simulink model "zynq_pmsm_motor_control"  (R2019b)
settings: Solver=FixedStepDiscrete  StartTime=0.0  StopTime=5000  FixedStep=0.002  RelTol=1e-3  EnableMultiTasking=on
undefined symbols (not defined in the file): DiscIntNeverNeededParam
libraries: simulink x1, simulink_extras x1
settings Model: SimulationMode=external  ExtModeTrigDuration=200000  Creator=krecmich  LastModifiedBy=cernylu6
settings DataIOCC: LimitDataPoints=on  SaveFormat=Array
settings OptimizationCC: ExpressionDepthLimit=2147483647  LifeSpan=1  EfficientTunableParamExpr=on
settings DebuggingCC: UnderspecifiedInitializationDetection=Classic  MergeDetectMultiDrivingBlocksExec=none  SolverPrmCheckMsg=warning  StateNameClashWarn=warning  SFUnexpectedBacktrackingDiag=warning  SFNoUnconditionalDefaultTransitionDiag=warning  SFExecutionAtInitializationDiag=none  ArithmeticOperatorsInVariantConditions=warning
settings HardwareCC: ProdBitPerLong=64  ProdLargestAtomicFloat=None  ProdHWDeviceType=Intel->x86-64
settings ModelReferenceCC: PropagateSignalLabelsOutOfModel=off
settings SFSimCC: SimUseLocalCustomCode=off  MATLABDynamicMemAlloc=off  CustomCodeUndefinedFunction=UseInterfaceOnly
settings RTWCC: Description=Linux Embedded Coder  SystemTargetFile=ert_linux.tlc  MakeCommand="make_rtw OPT_OPTS=\"-O2 -ggdb -Wall\" CC=arm-linux-gnueabihf-gcc CPP=arm-linux-gnueabihf-gcc"  TemplateMakefile=ert_linux.tmf  RTWUseLocalCustomCode=off  CustomSource=zynq_3pmdrv1_mc.c
settings CodeAppCC: IgnoreCustomStorageClasses=off  CustomSymbolStrType=$N$R$M  StateflowObjectComments=on  InternalIdentifier=Classic
settings STFCustomTargetCC: TargetLangStandard=C99 (ISO)  ModelReferenceCompliant=off  CombineOutputUpdateFcns=on  ERTCustomFileBanners=on  RemoveResetFunc=on  MATLABClassNameForMDSCustomization=Simulink.SoftwareTarget.ERTCustomization  SystemTargetFile=ert_linux.tlc
settings ERTTargetCC: TargetLangStandard=C99 (ISO)  MultiwordLength=2048  ModelReferenceCompliant=off  ParMdlRefBuildCompliant=off  CompOptLevelCompliant=off  ConcurrentExecutionCompliant=off  SupportContinuousTime=on  SupportNonInlinedSFcns=on  ModelStepFunctionPrototypeControlCompliant=off  CPPClassGenCompliant=off  UseToolchainInfoCompliant=off  ExtMode=on  ExtModeMexArgs='192.168.136.74'  ERTCustomFileTemplate=ert_linux_file_process.tlc  ConvertIfToSwitch=off  SuppressUnreachableDefaultCases=off
settings ConfigComp: CovMetricSettings=dw  CovHtmlReporting=on  CovSaveCumulativeToWorkspaceVar=on  CovSaveSingleToWorkspaceVar=on  CovExternalEMLEnable=off

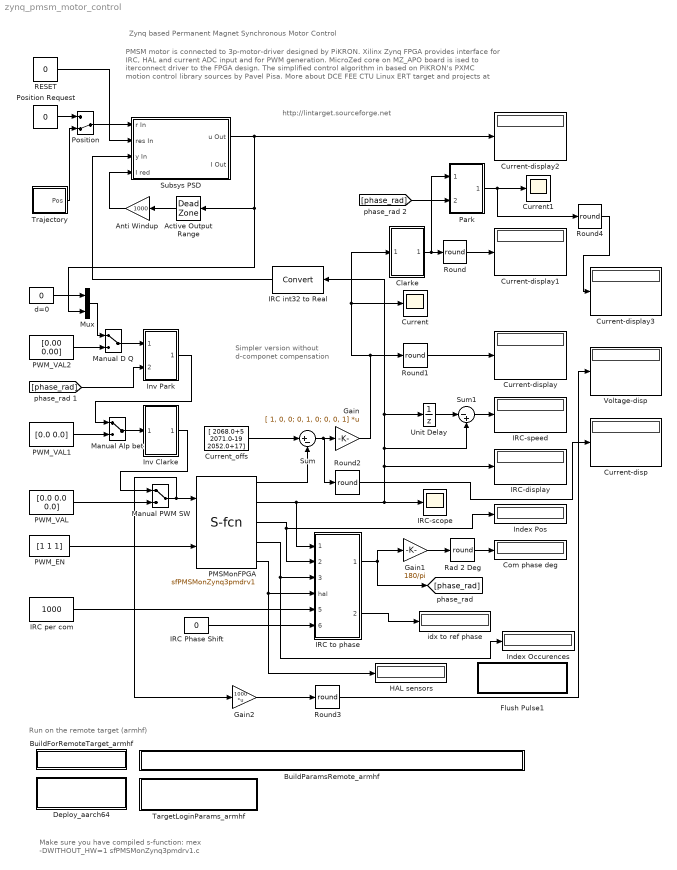
== system zynq_pmsm_motor_control ==
  note: Make sure you have compiled s-function:
      | mex -DWITHOUT_HW=1 sfPMSMonZynq3pmdrv1.c
  note: Simpler version without
      | d-componet compensation
  note: http://lintarget.sourceforge.net
  note: PMSM motor is connected to 3p-motor-driver designed by PiKRON. Xilinx Zynq FPGA provides
      | interface for  IRC, HAL and current ADC input and for PWM generation.
      | MicroZed core on MZ_APO board is ised to iterconnect driver to the FPGA design.
      | The simplified control algorithm in based on PiKRON's PXMC motion control
      | library sources by Pavel Pisa. More about DCE FEE CTU Linux ERT target and projects at
  note: Zynq based Permanent Magnet Synchronous Motor Control
  note: Run on the remote target (armhf)
  "  RESET" : Constant  Value=0
      settings: OpenFcn=if get_param(gcbh,'value')=='0' set_param(gcbh,'value','1'); else set_param(gcbh,'value','0'); end;
  Active Output Range : DeadZone  LowerValue=-0.8  UpperValue=0.8  LinearizeAsGain=off
  Anti Windup : Gain  Gain=1000
  BuildForRemoteTarget_armhf : Subsystem
      settings: OpenFcn=ert_linux_build(gcs, 'BuildParamsRemote_armhf')
      mask Display: disp('Build')
  BuildParamsRemote_armhf : Subsystem  mask{make_command='make_rtw OPT_OPTS="-O2 -ggdb -Wall" CC=arm-linux-gnueabihf-gcc CPP=arm-linux-gnueabihf-gcc'}
      mask prompts: make_command "MakeCommand"
      mask Display: disp(get_param(gcb, 'make_command'));
  Clarke : Subsystem
  Com phase deg : Display
  Current : Scope
  Current-disp : Display
  Current-display{,1..3} (4 alike) : Display
  Current1 : Scope
  Current_offs : Constant  Value="[ 2068.0+5  2071.0-19  2052.0+17]"
  Deploy_aarch64 : Subsystem
      settings: OpenFcn=ert_linux_deploy_and_connect(gcs, 'TargetLoginParams_armhf');
      mask Display: disp('Deploy and\nconnect')
  Flush Pulse1 : Subsystem  mask{target_ip_address='192.168.3.37'}
      mask prompts: target_ip_address "Target IP address"
      settings: OpenFcn=system(['./run_model_pmsm.sh ', get_param(bdroot(gcbh),'name'),' ', get_param(gcbh,'target_ip_address')]);
      mask Display: disp('Double Click\n to run model on Zynq')
  Gain : Gain  Gain=[ 1, 0, 0; 0, 1, 0; 0, 0, 1]  Multiplication=Matrix(K*u)
  Gain1 : Gain  Gain=180/pi
  Gain2 : Gain  Gain=1000  Multiplication=Matrix(K*u)
  HAL sensors : Display
  IRC Phase Shift : Constant  Value=0
  IRC int32 to Real : DataTypeConversion
  IRC per com : Constant  Value=1000  OutDataTypeStr=uint32
  IRC to phase : Subsystem
  IRC-display : Display
  IRC-scope : Scope
  IRC-speed : Display
  Index Occurences : Display
  Index Pos : Display
  Inv Clarke : Subsystem
  Inv Park : Subsystem
  Manual Alp bet : ManualSwitch
  Manual D Q : ManualSwitch
  Manual PWM SW : ManualSwitch
  Mux : Mux  Inputs=2
  PMSMonFPGA : S-Function  FunctionName=sfPMSMonZynq3pmdrv1  Parameters=Ts  SFunctionDeploymentMode=off  EnableBusSupport=off  mask{Ts=0.002}
      mask prompts: Ts "Sampling period (Ts):"
  PWM_EN : Constant  Value=[1 1 1]
  PWM_VAL : Constant  Value=[0.0 0.0 0.0]
  PWM_VAL1 : Constant  Value=[0.0 0.0]
  PWM_VAL2 : Constant  Value=[0.00 0.00]
  Park : Subsystem
  Position : ManualSwitch  CurrentSetting=0
  Position Request : Constant  Value=0
  Rad 2 Deg : Rounding  Operator=round
  Round{,1..4} (5 alike) : Rounding  Operator=round
  Subsys PSD : Subsystem  mask(optimized PSD controller){P=0.0006, I=0.002, D=0.001, Ts=0.002}
      mask prompts: P "P proportional (P):"; I "I integral (I):"; D "D derivative (D):"; Ts "Sampling period (Ts):"
      mask help:
      | Type: Subsystem block.
      |
      | Description:
      |   Subsystem covers optimized PSD controller (PSD represents discretized PID).
      |
      | Requirements:
      |   Sampling period Ts.
      mask Help:
      | <b>Type:</b> Subsystem block.
      | <br><br>
      | <b>Description:</b><br>
      |   Subsystem covers optimized PSD controller (PSD represents discretized PID).
      | <br><br>
      | <b>Requirements:</b><br>
      |   Sampling period Ts.
      mask Display:
      | color('orange');disp('\n          Opt. PSD\n          Controller');
      | color('green');port_label('input', 1, 'w');
      | color('red');port_label('input', 2, ' RSTs');
      | color('lightblue');port_label('input', 3, 'r');
      | color('orange');port_label('input', 4, 'red I');
      | color('orange');port_label('output', 1, 'u ');
      | color('orange');port_label('output', 2, 'I  ');
      | color('red');disp('\n\n\n\n\n\n\n       P');
  Sum : Sum  Inputs=|+-
  Sum1 : Sum  Inputs=|-+
  TargetLoginParams_armhf : Subsystem  mask{trgt_ip_addr='192.168.136.74', trgt_username='root'}
      mask prompts: trgt_ip_addr "Target IP address"; trgt_username "Target username"
      mask Display:
      | ip_addr = get_param(gcb, 'trgt_ip_addr');
      | user = get_param(gcb, 'trgt_username');
      | 
      | fprintf('IP addr:\t %s\n User:\t %s ', ip_addr, user);
  Trajectory : Subsystem
  Unit Delay : UnitDelay  SampleTime=-1  HasFrameUpgradeWarning=on
  Voltage-disp : Display
  d=0 : Constant  Value=0
  idx to ref phase : Display
  wires:
  Subsys PSD/1(u Out) -> Mux/2, Active Output Range/1, Current-display2/1
  "  RESET"/1 -> Subsys PSD/2(res In)
  Active Output Range/1 -> Anti Windup/1
  Anti Windup/1 -> Subsys PSD/4(I red)
  Position/1 -> Subsys PSD/1(r In)
  Position Request/1 -> Position/1
  Trajectory/1(Pos) -> Position/2
  PMSMonFPGA/2 -> IRC-scope/1, Unit Delay/1, IRC int32 to Real/1, Sum1/2, IRC-display/1, IRC to phase/1(irc_val)
  PWM_EN/1 -> PMSMonFPGA/2
  Round1/1 -> Current-display/1
  Current_offs/1 -> Sum/1
  Gain/1 -> Clarke/1("a, b, c"), Current/1, Round1/1
  PWM_VAL/1 -> Manual PWM SW/2
  Manual PWM SW/1 -> Gain2/1, PMSMonFPGA/1
  Round/1 -> Current-display1/1
  Clarke/1("alp, bet") -> Park/1("alp, bet"), Round/1
  PWM_VAL1/1 -> Manual Alp bet/2
  Manual Alp bet/1 -> Inv Clarke/1(alp,bet)
  Inv Clarke/1(a,b,c) -> Manual PWM SW/1
  Inv Park/1(alp,bet) -> Manual Alp bet/1
  Manual D Q/1 -> Inv Park/1(d,q)
  PWM_VAL2/1 -> Manual D Q/2
  Mux/1 -> Manual D Q/1
  d=0/1 -> Mux/1
  IRC to phase/1(phase rad) -> Gain1/1, [phase_rad]
  [phase_rad] -> Inv Park/2(angle rad)
  Gain1/1 -> Rad 2 Deg/1
  Rad 2 Deg/1 -> Com phase deg/1
  PMSMonFPGA/5 -> HAL sensors/1, IRC to phase/4(hal)
  IRC per com/1 -> IRC to phase/5(irc_per_com)
  PMSMonFPGA/3 -> Index Pos/1, IRC to phase/2(irc_indx)
  PMSMonFPGA/4 -> IRC to phase/3(irc_occur), Index Occurences/1
  [phase_rad] -> Park/2(angle rad)
  Park/1("d, q") -> Round4/1, Current1/1
  Unit Delay/1 -> Sum1/1
  Sum1/1 -> IRC-speed/1
  IRC int32 to Real/1 -> Subsys PSD/3(y In)
  IRC Phase Shift/1 -> IRC to phase/6(irc_ph_shift)
  Round2/1 -> Current-disp/1
  Gain2/1 -> Round3/1
  Round3/1 -> Voltage-disp/1
  Sum/1 -> Round2/1, Gain/1
  Round4/1 -> Current-display3/1
  PMSMonFPGA/1 -> Sum/2
  IRC to phase/2(idx to ref phase) -> idx to ref phase/1

== system zynq_pmsm_motor_control/BuildForRemoteTarget_armhf ==

== system zynq_pmsm_motor_control/BuildParamsRemote_armhf ==

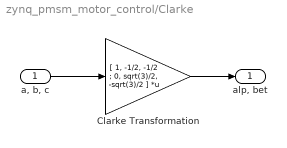
== system zynq_pmsm_motor_control/Clarke ==
  "a, b, c" : Inport
  Clarke Transformation : Gain  Gain=[ 1, -1/2, -1/2 ; 0, sqrt(3)/2, -sqrt(3)/2 ]  Multiplication=Matrix(K*u)
  "alp, bet" : Outport
  wires:
  "a, b, c"/1 -> Clarke Transformation/1
  Clarke Transformation/1 -> "alp, bet"/1

== system zynq_pmsm_motor_control/Deploy_aarch64 ==

== system zynq_pmsm_motor_control/Flush Pulse1 ==

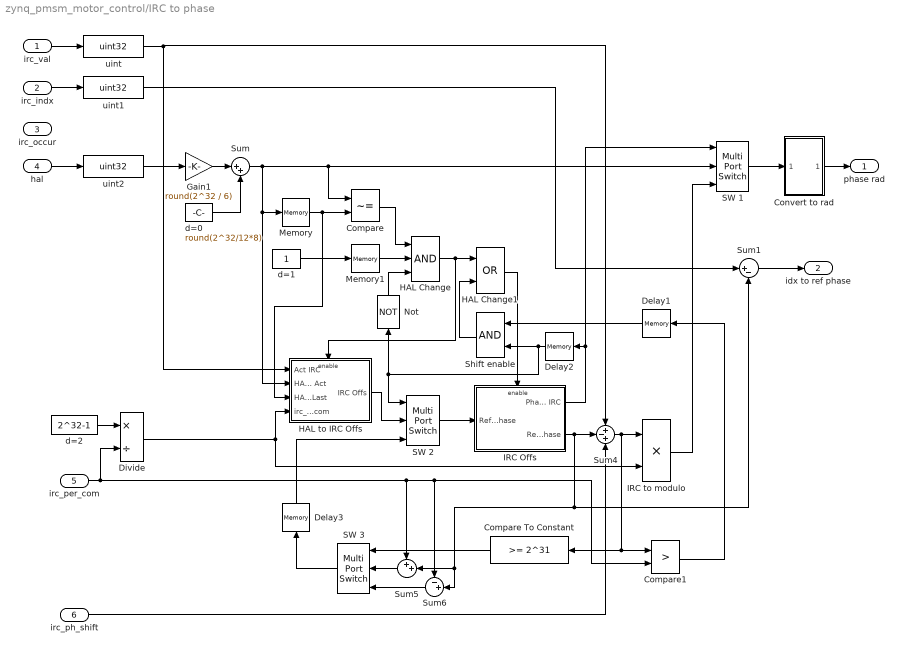
== system zynq_pmsm_motor_control/IRC to phase ==
  irc_val : Inport
  irc_indx : Inport  Port=2
  irc_occur : Inport  Port=3
  hal : Inport  Port=4
  irc_per_com : Inport  Port=5
  irc_ph_shift : Inport  Port=6
  Compare : RelationalOperator  Operator=~=  OutDataTypeStr=boolean  RndMeth=Nearest  InputSameDT=on
  Compare To Constant : simulink/Logic and Bit Operations/Compare To Constant  relop=>=  const=2^31  OutDataTypeStr=boolean
  Compare1 : RelationalOperator  Operator=>  OutDataTypeStr=boolean  RndMeth=Nearest  InputSameDT=on
  Convert to rad : Subsystem
  Delay1 : Memory
  Delay2 : Memory
  Delay3 : Memory
  Divide : Product  Inputs=*/  OutDataTypeStr=uint32
  Gain1 : Gain  Gain=round(2^32 / 6)  OutDataTypeStr=uint32
  HAL Change : Logic  Inputs=3  AllPortsSameDT=off  OutDataTypeStr=boolean
  HAL Change1 : Logic  Operator=OR  AllPortsSameDT=off  OutDataTypeStr=boolean
  HAL to IRC Offs : Subsystem
  IRC Offs : Subsystem  TreatAsAtomicUnit=on
  IRC to modulo : Product  OutDataTypeStr=uint32
  Memory : Memory
  Memory1 : Memory
  Not : Logic  Operator=NOT  Inputs=1  AllPortsSameDT=off  OutDataTypeStr=boolean
  SW 1 : MultiPortSwitch  DataPortOrder=Zero-based contiguous  Inputs=2  zeroidx=on  OutDataTypeStr=uint32
  SW 2 : MultiPortSwitch  DataPortOrder=Zero-based contiguous  Inputs=2  zeroidx=on  OutDataTypeStr=uint32
  SW 3 : MultiPortSwitch  DataPortOrder=Zero-based contiguous  Inputs=2  zeroidx=on  OutDataTypeStr=uint32
  Shift enable : Logic  AllPortsSameDT=off  OutDataTypeStr=boolean
  Sum : Sum  Inputs=|++  AccumDataTypeStr=uint32  OutDataTypeStr=uint32
  Sum1 : Sum  Inputs=|+-  AccumDataTypeStr=int32  OutDataTypeStr=uint32
  Sum4 : Sum  Inputs=+-+  AccumDataTypeStr=int32  OutDataTypeStr=uint32
  Sum5 : Sum  Inputs=++|  AccumDataTypeStr=int32  OutDataTypeStr=uint32
  Sum6 : Sum  Inputs=-+|  AccumDataTypeStr=int32  OutDataTypeStr=uint32
  d=0 : Constant  Value=round(2^32/12*8)  OutDataTypeStr=uint32
  d=1 : Constant  OutDataTypeStr=boolean
  d=2 : Constant  Value=2^32-1  OutDataTypeStr=uint32
  uint : DataTypeConversion  OutDataTypeStr=uint32  RndMeth=Simplest
  uint1 : DataTypeConversion  OutDataTypeStr=uint32  RndMeth=Simplest
  uint2 : DataTypeConversion  OutDataTypeStr=uint32  RndMeth=Simplest
  phase rad : Outport
  idx to ref phase : Outport  Port=2
  wires:
  irc_val/1 -> uint/1
  irc_indx/1 -> uint1/1
  hal/1 -> uint2/1
  uint2/1 -> Gain1/1
  Gain1/1 -> Sum/1
  d=0/1 -> Sum/2
  Memory/1 -> HAL to IRC Offs/3(HAL Ph Last), Compare/2
  SW 1/1 -> Convert to rad/1(uint32)
  Convert to rad/1(rad) -> phase rad/1
  Sum/1 -> HAL to IRC Offs/2(HAL Ph Act), Memory/1, Compare/1, SW 1/2
  d=1/1 -> Memory1/1
  Memory1/1 -> HAL Change/2
  Compare/1 -> HAL Change/1
  uint/1 -> HAL to IRC Offs/1(Act IRC), Sum4/1
  IRC Offs/2(Reg ref phase) -> Sum1/2, Sum5/2, Sum6/2, Sum4/2
  Not/1 -> HAL Change/3
  IRC Offs/1(Phase by IRC) -> SW 1/1, Delay2/1
  SW 2/1 -> IRC Offs/1(Ref phase)
  HAL Change/1 -> HAL Change1/1, HAL to IRC Offs/Enable
  HAL Change1/1 -> IRC Offs/Enable
  Sum4/1 -> Compare1/1, Compare To Constant/1, IRC to modulo/1
  IRC to modulo/1 -> SW 1/3
  Compare To Constant/1 -> SW 3/1
  Sum5/1 -> SW 3/2
  Sum6/1 -> SW 3/3
  Compare1/1 -> Delay1/1
  Delay2/1 -> Shift enable/2, SW 2/1, Not/1
  Delay3/1 -> SW 2/3
  SW 3/1 -> Delay3/1
  d=2/1 -> Divide/1
  irc_per_com/1 -> Divide/2, Sum5/1, Compare1/2, Sum6/1
  Divide/1 -> HAL to IRC Offs/4(irc_per_com), IRC to modulo/2
  HAL to IRC Offs/1(IRC Offs) -> SW 2/2
  irc_ph_shift/1 -> Sum4/3
  Delay1/1 -> Shift enable/1
  Shift enable/1 -> HAL Change1/2
  uint1/1 -> Sum1/1
  Sum1/1 -> idx to ref phase/1

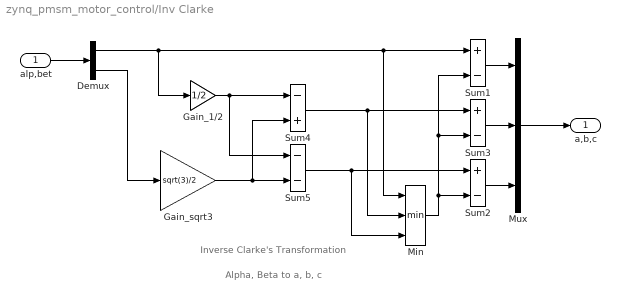
== system zynq_pmsm_motor_control/Inv Clarke ==
  note: Inverse Clarke's Transformation
  note: Alpha, Beta to a, b, c
  alp,bet : Inport
  Demux : Demux  Outputs=2
  Gain_1/2 : Gain  Gain=1/2
  Gain_sqrt3 : Gain  Gain=sqrt(3)/2
  Min : MinMax  Inputs=3
  Mux : Mux  Inputs=3
  Sum1 : Sum  Inputs=+-
  Sum2 : Sum  Inputs=+-
  Sum3 : Sum  Inputs=+-
  Sum4 : Sum  Inputs=-+
  Sum5 : Sum  Inputs=--
  a,b,c : Outport
  wires:
  alp,bet/1 -> Demux/1
  Mux/1 -> a,b,c/1
  Sum2/1 -> Mux/3
  Sum1/1 -> Mux/1
  Sum3/1 -> Mux/2
  Min/1 -> Sum3/2, Sum1/2, Sum2/2
  Demux/1 -> Gain_1/2/1, Min/1, Sum1/1
  Demux/2 -> Gain_sqrt3/1
  Gain_1/2/1 -> Sum5/1, Sum4/1
  Gain_sqrt3/1 -> Sum5/2, Sum4/2
  Sum4/1 -> Min/2, Sum3/1
  Sum5/1 -> Min/3, Sum2/1

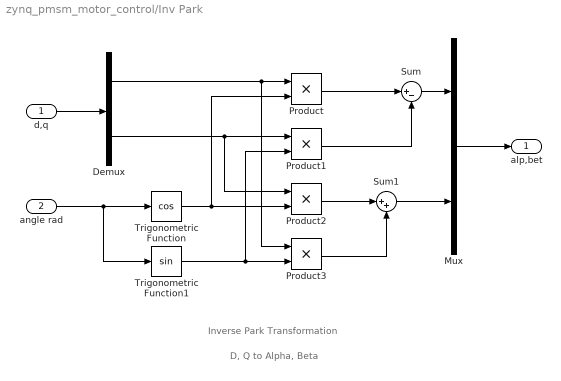
== system zynq_pmsm_motor_control/Inv Park ==
  note: D, Q to Alpha, Beta
  note: Inverse Park Transformation
  d,q : Inport
  angle rad : Inport  Port=2
  Demux : Demux  Outputs=2
  Mux : Mux  Inputs=2
  Product{,1..3} (4 alike) : Product
  Sum : Sum  Inputs=|+-
  Sum1 : Sum  Inputs=|++
  Trigonometric Function : Trigonometry  Operator=cos
  Trigonometric Function1 : Trigonometry
  alp,bet : Outport
  wires:
  Mux/1 -> alp,bet/1
  d,q/1 -> Demux/1
  Product/1 -> Sum/1
  Demux/1 -> Product3/1, Product/1
  Trigonometric Function/1 -> Product/2, Product2/2
  Sum/1 -> Mux/1
  Sum1/1 -> Mux/2
  Product1/1 -> Sum/2
  Demux/2 -> Product2/1, Product1/1
  Trigonometric Function1/1 -> Product3/2, Product1/2
  Product2/1 -> Sum1/1
  Product3/1 -> Sum1/2
  angle rad/1 -> Trigonometric Function1/1, Trigonometric Function/1

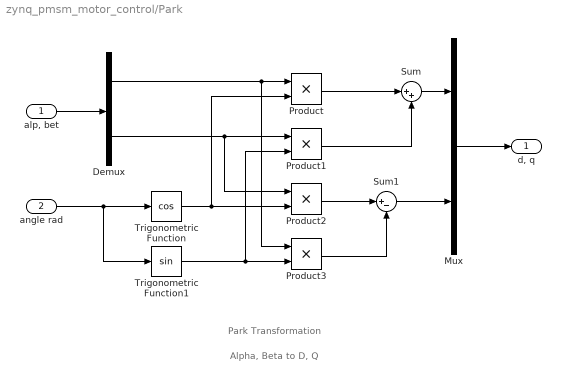
== system zynq_pmsm_motor_control/Park ==
  note: Alpha, Beta to D, Q
  note: Park Transformation
  "alp, bet" : Inport
  angle rad : Inport  Port=2
  Demux : Demux  Outputs=2
  Mux : Mux  Inputs=2
  Product{,1..3} (4 alike) : Product
  Sum : Sum  Inputs=|++
  Sum1 : Sum  Inputs=|+-
  Trigonometric Function : Trigonometry  Operator=cos
  Trigonometric Function1 : Trigonometry
  "d, q" : Outport
  wires:
  Mux/1 -> "d, q"/1
  "alp, bet"/1 -> Demux/1
  Product/1 -> Sum/1
  Demux/1 -> Product3/1, Product/1
  Trigonometric Function/1 -> Product/2, Product2/2
  Sum/1 -> Mux/1
  Sum1/1 -> Mux/2
  Product1/1 -> Sum/2
  Demux/2 -> Product2/1, Product1/1
  Trigonometric Function1/1 -> Product3/2, Product1/2
  Product2/1 -> Sum1/1
  Product3/1 -> Sum1/2
  angle rad/1 -> Trigonometric Function1/1, Trigonometric Function/1

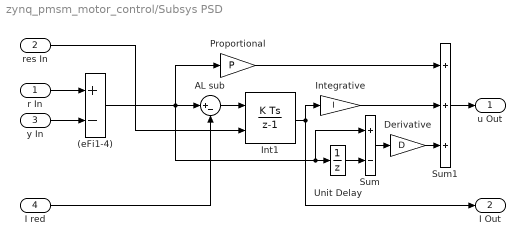
== system zynq_pmsm_motor_control/Subsys PSD ==
  r In : Inport  SampleTime=Ts
  res In : Inport  Port=2
  y In : Inport  Port=3  SampleTime=Ts
  I red : Inport  Port=4
  "  Derivative" : Gain  Gain=D  SaturateOnIntegerOverflow=on  OutDataTypeStr=Inherit: Same as input  ParamDataTypeStr=Inherit: Same as input
  (eFi1-4) : Sum  Inputs=+-  SaturateOnIntegerOverflow=on  InputSameDT=on  OutDataTypeStr=Inherit: Same as first input
  AL sub : Sum  Inputs=|+-  SaturateOnIntegerOverflow=on  InputSameDT=on  OutDataTypeStr=Inherit: Same as first input
  Int1 : DiscreteIntegrator  ExternalReset=level  SampleTime=-1  ICPrevOutput=DiscIntNeverNeededParam  ICPrevScaledInput=DiscIntNeverNeededParam
  Integrative : Gain  Gain=I  SaturateOnIntegerOverflow=on  OutDataTypeStr=Inherit: Same as input  ParamDataTypeStr=Inherit: Same as input
  Proportional : Gain  Gain=P  SaturateOnIntegerOverflow=on  OutDataTypeStr=Inherit: Same as input  ParamDataTypeStr=Inherit: Same as input
  Sum : Sum  Inputs=+-  SaturateOnIntegerOverflow=on  InputSameDT=on  OutDataTypeStr=Inherit: Same as first input
  Sum1 : Sum  Inputs=+++  SaturateOnIntegerOverflow=on  InputSameDT=on  OutDataTypeStr=Inherit: Same as first input
  Unit Delay : UnitDelay  SampleTime=Ts  HasFrameUpgradeWarning=on
  u Out : Outport
  I Out : Outport  Port=2
  wires:
  r In/1 -> (eFi1-4)/1
  y In/1 -> (eFi1-4)/2
  (eFi1-4)/1 -> Proportional/1, AL sub/1, Sum/1, Unit Delay/1
  "  Derivative"/1 -> Sum1/3
  Int1/1 -> I Out/1, Integrative/1
  Proportional/1 -> Sum1/1
  Sum1/1 -> u Out/1
  Sum/1 -> "  Derivative"/1
  Unit Delay/1 -> Sum/2
  res In/1 -> Int1/2
  AL sub/1 -> Int1/1
  I red/1 -> AL sub/2
  Integrative/1 -> Sum1/2

== system zynq_pmsm_motor_control/TargetLoginParams_armhf ==

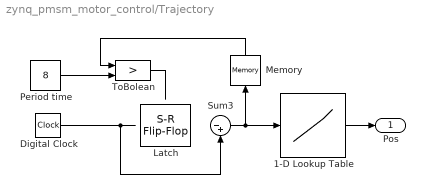
== system zynq_pmsm_motor_control/Trajectory ==
  1-D Lookup Table : Lookup_n-D  NumberOfTableDimensions=1  BreakpointsForDimension1="[0 3      5     6     6.1 8]"  Table="[0 2000 500 500 0    0]"  RndMeth=Simplest  InputSameDT=on
  Digital Clock : DigitalClock  SampleTime=0.002
  Latch : simulink_extras/Flip Flops/S-R Flip-Flop  initial_condition=0
  Memory : Memory
  Period time : Constant  Value=8
  Sum3 : Sum  Inputs=|-+  SaturateOnIntegerOverflow=on  InputSameDT=on  OutDataTypeStr=Inherit: Same as first input
  ToBolean : RelationalOperator  Operator=>  RndMeth=Nearest
  Pos : Outport
  wires:
  Digital Clock/1 -> Sum3/2
  Sum3/1 -> 1-D Lookup Table/1, Memory/1
  1-D Lookup Table/1 -> Pos/1
  ? -> Sum3/1
  ToBolean/1 -> ?
  Period time/1 -> ToBolean/2
  Memory/1 -> ToBolean/1

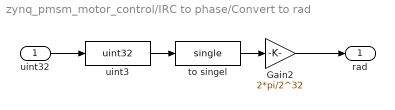
== system zynq_pmsm_motor_control/IRC to phase/Convert to rad ==
  uint32 : Inport
  Gain2 : Gain  Gain=2*pi/2^32  OutDataTypeStr=single
  to singel : DataTypeConversion  OutDataTypeStr=single  RndMeth=Simplest
  uint3 : DataTypeConversion  OutDataTypeStr=uint32  RndMeth=Simplest
  rad : Outport
  wires:
  uint3/1 -> to singel/1
  Gain2/1 -> rad/1
  to singel/1 -> Gain2/1
  uint32/1 -> uint3/1

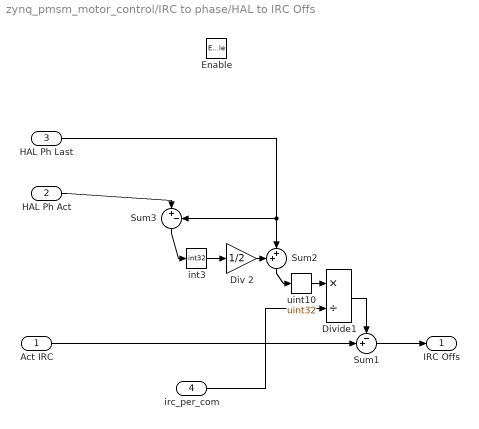
== system zynq_pmsm_motor_control/IRC to phase/HAL to IRC Offs ==
  Act IRC : Inport
  HAL Ph Act : Inport  Port=2
  HAL Ph Last : Inport  Port=3
  irc_per_com : Inport  Port=4
  Enable : EnablePort
  Div 2 : Gain  Gain=1/2  OutDataTypeStr=int32
  Divide1 : Product  Inputs=*/  OutDataTypeStr=uint32
  Sum1 : Sum  Inputs=-+|  AccumDataTypeStr=uint32  OutDataTypeStr=uint32
  Sum2 : Sum  Inputs=++|  AccumDataTypeStr=uint32  OutDataTypeStr=uint32
  Sum3 : Sum  Inputs=|+-  AccumDataTypeStr=int32  OutDataTypeStr=uint32
  int3 : DataTypeConversion  OutDataTypeStr=int32  RndMeth=Simplest
  uint10 : DataTypeConversion  OutDataTypeStr=uint32  RndMeth=Simplest
  IRC Offs : Outport
  wires:
  irc_per_com/1 -> Divide1/2
  HAL Ph Last/1 -> Sum2/2, Sum3/2
  Div 2/1 -> Sum2/1
  int3/1 -> Div 2/1
  Sum3/1 -> int3/1
  Sum1/1 -> IRC Offs/1
  Divide1/1 -> Sum1/1
  uint10/1 -> Divide1/1
  Sum2/1 -> uint10/1
  Act IRC/1 -> Sum1/2
  HAL Ph Act/1 -> Sum3/1

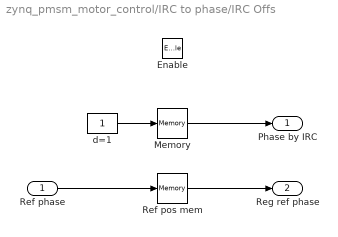
== system zynq_pmsm_motor_control/IRC to phase/IRC Offs ==
  Ref phase : Inport
  Enable : EnablePort
  Memory : Memory  InheritSampleTime=on
  Ref pos mem : Memory  InheritSampleTime=on
  d=1 : Constant  OutDataTypeStr=uint32
  Phase by IRC : Outport
  Reg ref phase : Outport  Port=2
  wires:
  d=1/1 -> Memory/1
  Memory/1 -> Phase by IRC/1
  Ref pos mem/1 -> Reg ref phase/1
  Ref phase/1 -> Ref pos mem/1
